simulink model "pendulum_adrc_sim"  (R2025b)
settings: Solver=VariableStepAuto  StartTime=0.0  StopTime=Tsim  RelTol=rel_tol
undefined symbols (not defined in the file): A, B, b0, C, c, g, k1, k2, L, l, M, manual_control_flag, pow, theta_dot_init, theta_init, theta_setpoint, Ts, u_manual
libraries: simulink x1
settings Model: Creator=michele.schiavo

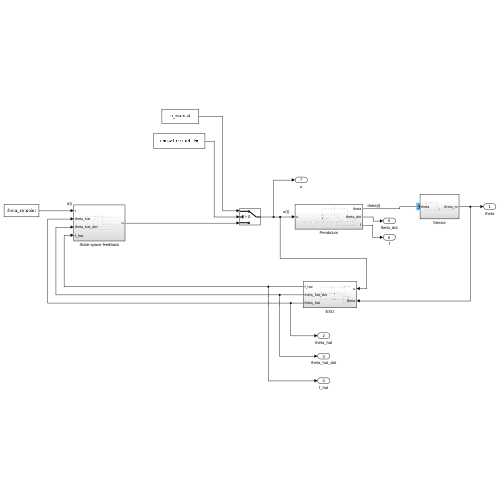
[thumbnail: Simulink's stored preview of the top-level diagram]
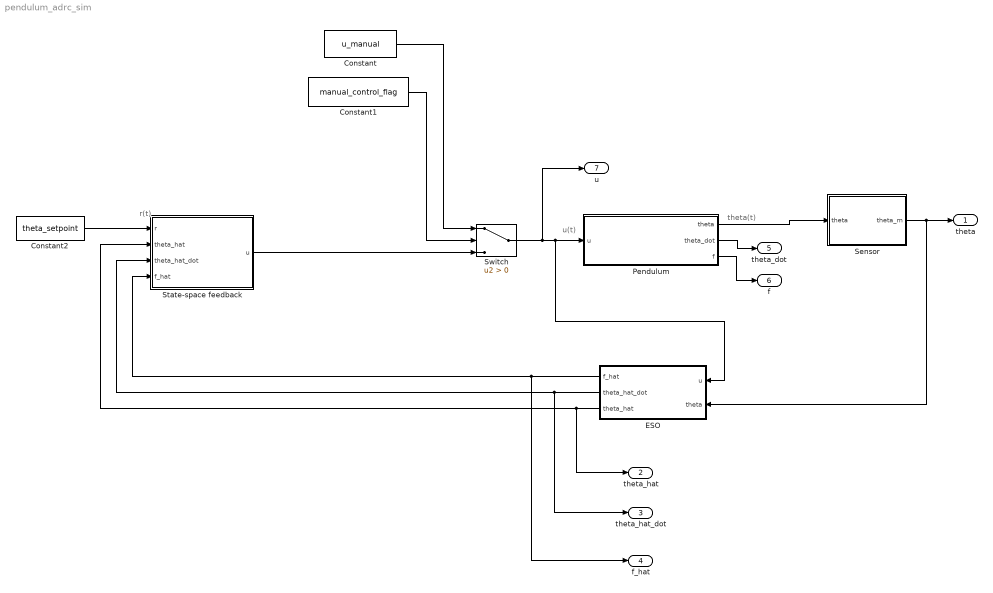
== system pendulum_adrc_sim ==
  note: r(t)
  note: u(t)
  note: theta(t)
  Constant : Constant  Value=u_manual
  Constant1 : Constant  Value=manual_control_flag
  Constant2 : Constant  Value=theta_setpoint
  ESO : Subsystem
  Pendulum : Subsystem
  Sensor : Subsystem
  State-space feedback : Subsystem
  Switch : Switch  Criteria=u2 > Threshold  SaturateOnIntegerOverflow=off  InputSameDT=off
  theta : Outport
  theta_hat : Outport  Port=2
  theta_hat_dot : Outport  Port=3
  f_hat : Outport  Port=4
  theta_dot : Outport  Port=5
  f : Outport  Port=6
  u : Outport  Port=7
  wires:
  Switch/1 -> u/1, ESO/1(u), Pendulum/1(u)
  Constant/1 -> Switch/1
  Constant1/1 -> Switch/2
  Constant2/1 -> State-space feedback/1(r)
  State-space feedback/1(u) -> Switch/3
  ESO/1(f_hat) -> f_hat/1, State-space feedback/4(f_hat)
  ESO/2(theta_hat_dot) -> theta_hat_dot/1, State-space feedback/3(theta_hat_dot)
  ESO/3(theta_hat) -> theta_hat/1, State-space feedback/2(theta_hat)
  Pendulum/2(theta_dot) -> theta_dot/1
  Pendulum/3(f) -> f/1
  Pendulum/1(theta) -> Sensor/1(theta)
  Sensor/1(theta_m) -> ESO/2(theta), theta/1

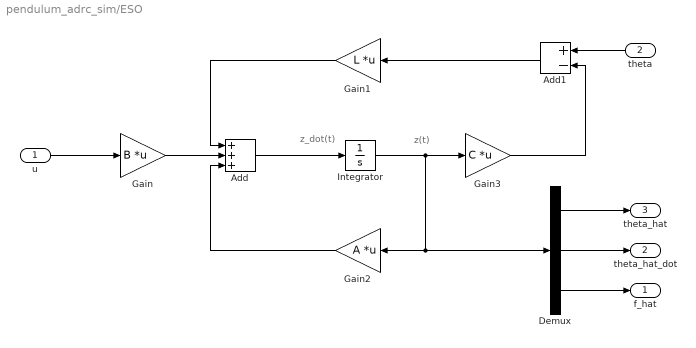
== system pendulum_adrc_sim/ESO ==
  note: z(t)
  note: z_dot(t)
  u : Inport
  theta : Inport  Port=2
  Add : Sum  Inputs=+++
  Add1 : Sum  Inputs=+-
  Demux : Demux  Outputs=3
  Gain : Gain  Gain=B  Multiplication=Matrix(K*u)
  Gain1 : Gain  Gain=L  Multiplication=Matrix(K*u)
  Gain2 : Gain  Gain=A  Multiplication=Matrix(K*u)
  Gain3 : Gain  Gain=C  Multiplication=Matrix(K*u)
  Integrator : Integrator
  f_hat : Outport
  theta_hat_dot : Outport  Port=2
  theta_hat : Outport  Port=3
  wires:
  Gain3/1 -> Add1/2
  Add/1 -> Integrator/1
  Gain2/1 -> Add/3
  Gain/1 -> Add/2
  Gain1/1 -> Add/1
  Integrator/1 -> Demux/1, Gain2/1, Gain3/1
  Add1/1 -> Gain1/1
  u/1 -> Gain/1
  theta/1 -> Add1/1
  Demux/3 -> f_hat/1
  Demux/2 -> theta_hat_dot/1
  Demux/1 -> theta_hat/1

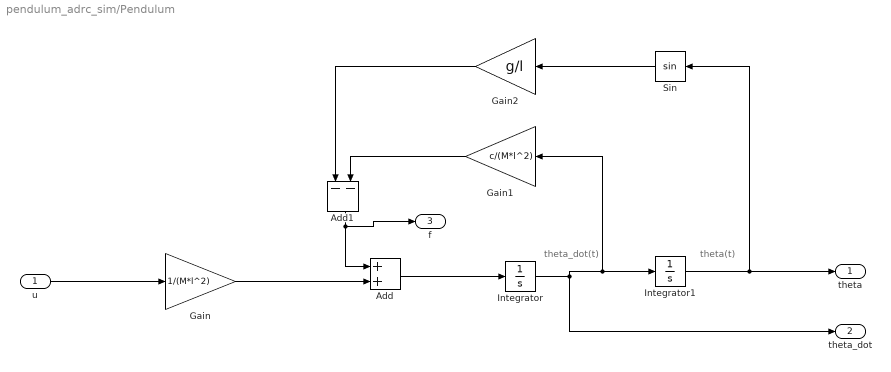
== system pendulum_adrc_sim/Pendulum ==
  note: theta(t)
  note: theta_dot(t)
  u : Inport
  Add : Sum
  Add1 : Sum  Inputs=--
  Gain : Gain  Gain=1/(M*l^2)
  Gain1 : Gain  Gain=c/(M*l^2)
  Gain2 : Gain  Gain=g/l
  Integrator : Integrator  InitialCondition=theta_dot_init
  Integrator1 : Integrator  InitialCondition=theta_init
  Sin : Trigonometry
  theta : Outport
  theta_dot : Outport  Port=2
  f : Outport  Port=3
  wires:
  Integrator1/1 -> theta/1, Sin/1
  Gain/1 -> Add/2
  u/1 -> Gain/1
  Integrator/1 -> Gain1/1, Integrator1/1, theta_dot/1
  Add/1 -> Integrator/1
  Sin/1 -> Gain2/1
  Add1/1 -> f/1, Add/1
  Gain1/1 -> Add1/2
  Gain2/1 -> Add1/1

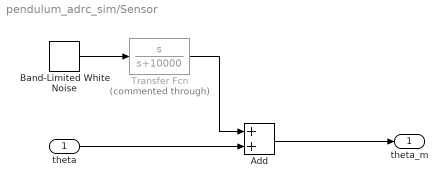
== system pendulum_adrc_sim/Sensor ==
  theta : Inport
  Add : Sum
  Band-Limited White Noise : simulink/Sources/Band-Limited White Noise  Cov=[pow]  Ts=Ts  seed=[23341]
  Transfer Fcn : TransferFcn  Commented=through  Numerator=[1 0]  Denominator=[1 10000]
  theta_m : Outport
  wires:
  Transfer Fcn/1 -> Add/1
  theta/1 -> Add/2
  Add/1 -> theta_m/1
  Band-Limited White Noise/1 -> Transfer Fcn/1

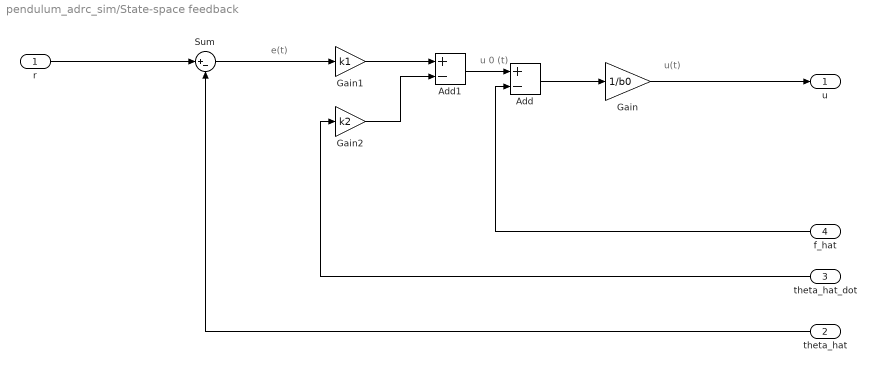
== system pendulum_adrc_sim/State-space feedback ==
  note: u 0 (t)
  note: e(t)
  note: u(t)
  r : Inport
  theta_hat : Inport  Port=2
  theta_hat_dot : Inport  Port=3
  f_hat : Inport  Port=4
  Add : Sum  Inputs=+-
  Add1 : Sum  Inputs=+-
  Gain : Gain  Gain=1/b0
  Gain1 : Gain  Gain=k1
  Gain2 : Gain  Gain=k2
  Sum : Sum  Inputs=|+-
  u : Outport
  wires:
  Sum/1 -> Gain1/1
  r/1 -> Sum/1
  Gain1/1 -> Add1/1
  Add1/1 -> Add/1
  Add/1 -> Gain/1
  Gain2/1 -> Add1/2
  Gain/1 -> u/1
  f_hat/1 -> Add/2
  theta_hat_dot/1 -> Gain2/1
  theta_hat/1 -> Sum/2
